simulink library "Yaw_Motor_Lib_org"  (Simulink 10.0)
settings: Solver=ode45  StartTime=0.0  StopTime=10.0  RelTol=1e-3  EnableMultiTasking=on
undefined symbols (not defined in the file): WT_Params
libraries: fl_lib x6, nesl_utility x5, elec_lib x1, sdl_lib x1, Yaw_Gearbox_Lib x1
Description:
  | Copyright 2009-2017 The MathWorks, Inc. MathWorks, Inc.
settings Model: Creator=smiller  LastModifiedBy=annonymous

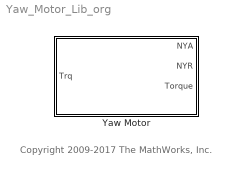
== system Yaw_Motor_Lib_org ==
  note: Copyright 2009-2017 The MathWorks, Inc.
  Yaw Motor : Subsystem
      mask Display: image(imread('Yaw_Servomotor_Horizontal_IMAGE.jpg'));

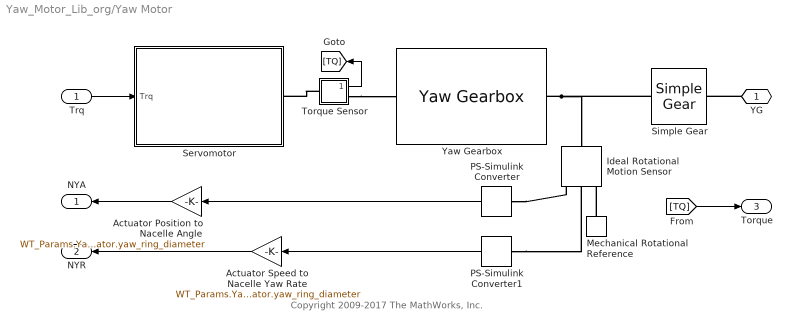
== system Yaw_Motor_Lib_org/Yaw Motor ==
  note: Copyright 2009-2017 The MathWorks, Inc.
  Trq : Inport
  Actuator Position to Nacelle Angle : Gain  Gain=WT_Params.Yaw_Actuator.yaw_gear_diameter/WT_Params.Yaw_Actuator.yaw_ring_diameter
  Actuator Speed to Nacelle Yaw Rate : Gain  Gain=WT_Params.Yaw_Actuator.yaw_gear_diameter/WT_Params.Yaw_Actuator.yaw_ring_diameter
  Ideal Rotational Motion Sensor : fl_lib/Mechanical/Mechanical Sensors/Ideal Rotational Motion Sensor  offset=0 rad
  Mechanical Rotational Reference : fl_lib/Mechanical/Rotational Elements/Mechanical Rotational Reference
  PS-Simulink Converter : nesl_utility/PS-Simulink Converter  PhysicalDomain=network_engine_domain  SubClassName=ps_output  LeftPortType=input  RightPortType=output  PseudoPeriodic=off  Frequencies=[]  Unit=deg  AffineConversion=off
  PS-Simulink Converter1 : nesl_utility/PS-Simulink Converter  PhysicalDomain=network_engine_domain  SubClassName=ps_output  LeftPortType=input  RightPortType=output  PseudoPeriodic=off  Frequencies=[]  Unit=deg/s  AffineConversion=off
  Servomotor : Subsystem
      mask Display: image(imread('Yaw_Servomotor_IMAGE.jpg'));
  Simple Gear : sdl_lib/Gears/Simple Gear  ratio=1/(WT_Params.Yaw_Actuator.yaw_gear_diameter/WT_Params.Yaw_Actuator.yaw_ring_diameter)  rotation_direction=2  friction_model=1  T_noload=0.1 N*m  T_nom=5 N*m  efficiency_nom=0.8  efficiency=0.8  mu_visc=[ 0 0 ] N*m/(rad/s)  w_thr=0.01 rad/s  pwr_thr=0.001 W  enable_faults=simscape.enum.onoff.off  efficiency_fault=0.05  external_fault=simscape.enum.onoff.off  temporal_fault=simscape.enum.onoff.off  fault_time=5 s  fault_angles=pi / 12 rad  report_fault=1  temperature_TLU=[ 280 300 320 ] K  load_TLU=[ 1 5 10 ] N*m  efficiency_TLU=[ 0.95 0.9 0.85 ]  efficiency_TLU2=[ 0.85 0.8 0.75; 0.95 0.9 0.85; 0.85 0.8 0.7 ]  thermal_mass=50 J/K  T_init=300 K
      settings: SourceProductName=Simscape Driveline
  Torque Sensor : Subsystem
      mask Display: disp('S')
  Yaw Gearbox : Yaw_Gearbox_Lib/Yaw Gearbox  SystemSampleTime=-1
  YG : PMIOPort  Side=Right
  NYA : Outport
  NYR : Outport  Port=2
  Torque : Outport  Port=3
  wires:
  PS-Simulink Converter1/1 -> Actuator Speed to Nacelle Yaw Rate/1
  PS-Simulink Converter/1 -> Actuator Position to Nacelle Angle/1
  [TQ] -> Torque/1
  Torque Sensor/1(Trq) -> [TQ]
  Actuator Speed to Nacelle Yaw Rate/1 -> NYR/1
  Actuator Position to Nacelle Angle/1 -> NYA/1
  Trq/1 -> Servomotor/1(Trq)
  connections:
  YG/RConn1 -- Simple Gear/RConn1
  PS-Simulink Converter/LConn1 -- Ideal Rotational Motion Sensor/RConn3
  Mechanical Rotational Reference/LConn1 -- Ideal Rotational Motion Sensor/RConn1
  PS-Simulink Converter1/LConn1 -- Ideal Rotational Motion Sensor/RConn2
  Yaw Gearbox/RConn1 -- Ideal Rotational Motion Sensor/LConn1 -- Simple Gear/LConn1
  Torque Sensor/RConn1 -- Yaw Gearbox/LConn1
  Torque Sensor/LConn1 -- Servomotor/RConn1

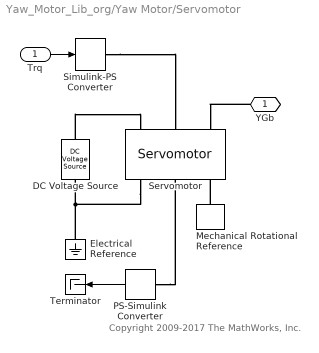
== system Yaw_Motor_Lib_org/Yaw Motor/Servomotor ==
  note: Copyright 2009-2017 The MathWorks, Inc.
  Trq : Inport
  DC Voltage Source : fl_lib/Electrical/Electrical Sources/DC Voltage Source  v0=WT_Params.Yaw_Actuator.Motor.voltage V
  Electrical Reference : fl_lib/Electrical/Electrical Elements/Electrical Reference
  Mechanical Rotational Reference : fl_lib/Mechanical/Rotational Elements/Mechanical Rotational Reference
  PS-Simulink Converter : nesl_utility/PS-Simulink Converter  PhysicalDomain=network_engine_domain  SubClassName=ps_output  LeftPortType=input  RightPortType=output  PseudoPeriodic=off  Frequencies=[]  Unit=deg/s  AffineConversion=off
  Servomotor : elec_lib/Actuators & Drivers/Rotational Actuators/Servomotor  torque_speed_param=1  w_t=WT_Params.Yaw_Actuator.Motor.max_speed_vector rpm  T_t=WT_Params.Yaw_Actuator.Motor.max_torque_vector N*m  torque_max=0.1 N*m  power_max=30 W  Tc=WT_Params.Yaw_Actuator.Motor.control_time_constant s  losses_param=1  eff=100  w_eff=3.75e+03 rpm  T_eff=0.08 N*m  Piron=0 W  Pbase=0 W  w_eff_vec=[-8000 -4000 0 4000 8000] rpm  T_eff_vec=[0 0.03 0.06 0.09] N*m  losses_mat=[1.49 1.67 2.21 3.10; 0.42 0.69 1.14 2.03; 0.06 0.24 0.78 1.68; 0.42 0.69 1.14 2.03; 1.49 1.67 2.21 3.10] W  efficiency_mat=[95 95 95 95; 95 95 95 95; 95 95 95 95; 95 95 95 95; 95 95 95 95]  Res=WT_Params.Yaw_Actuator.Motor.resistance Ohm  J=0 kg*m^2  lam=WT_Params.Yaw_Actuator.Motor.damping N*m/(rad/s)  speed0=0 rpm  alpha=0.00393 1/K  Tmeas=25 C  Tmeas2=125 C  losses_mat_T2=[1.49 1.74 2.49 3.74;0.42 0.67 1.42 2.67;0.06 0.31 1.06 2.31;0.42 0.67 1.42 2.67;1.49 1.74 2.49 3.74] W  efficiency_mat_T2=[95 95 95 95; 95 95 95 95; 95 95 95 95; 95 95 95 95; 95 95 95 95]  thermal_mass=100 J/K  initial_temperature=25 C  fault_condition=1  fault_threshold=0.5
      settings: SourceProductName=Simscape Electrical  SourceProductBaseCode=PS
  Simulink-PS Converter : nesl_utility/Simulink-PS Converter  PhysicalDomain=network_engine_domain  SubClassName=ps_input  LeftPortType=input  RightPortType=output  PseudoPeriodic=off  Frequencies=[]  NoiseDistribution=none  NoiseParameters=[]  Unit=1  AffineConversion=off  FilteringAndDerivatives=filter  SimscapeFilterOrder=1  InputFilterTimeConstant=WT_Params.Yaw_Actuator.Motor.filter_constant  UdotUserProvided=1
  Terminator : Terminator
  YGb : PMIOPort  Side=Right
  wires:
  Trq/1 -> Simulink-PS Converter/1
  PS-Simulink Converter/1 -> Terminator/1
  connections:
  YGb/RConn1 -- Servomotor/LConn3
  Simulink-PS Converter/RConn1 -- Servomotor/LConn2
  PS-Simulink Converter/LConn1 -- Servomotor/RConn2
  Mechanical Rotational Reference/LConn1 -- Servomotor/RConn3
  Electrical Reference/LConn1 -- DC Voltage Source/RConn1 -- Servomotor/RConn1
  DC Voltage Source/LConn1 -- Servomotor/LConn1

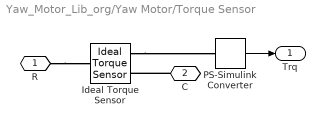
== system Yaw_Motor_Lib_org/Yaw Motor/Torque Sensor ==
  Ideal Torque Sensor : fl_lib/Mechanical/Mechanical Sensors/Ideal Torque Sensor
  PS-Simulink Converter : nesl_utility/PS-Simulink Converter  PhysicalDomain=network_engine_domain  SubClassName=ps_output  LeftPortType=input  RightPortType=output  PseudoPeriodic=off  Frequencies=[]  Unit=1  AffineConversion=off
  R : PMIOPort  Side=Left
  C : PMIOPort  Port=2  Side=Right
  Trq : Outport
  wires:
  PS-Simulink Converter/1 -> Trq/1
  connections:
  Ideal Torque Sensor/RConn2 -- PS-Simulink Converter/LConn1
  C/RConn1 -- Ideal Torque Sensor/RConn1
  R/RConn1 -- Ideal Torque Sensor/LConn1
